simulink model "road_disturbances"  (R2020b)
settings: Solver=VariableStepAuto  StartTime=0.0  StopTime=10.0  MaxStep=1e-2  RelTol=1e-3
libraries: simulink x2
settings Model: Creator=kjartan  LastModifiedBy=kjartan

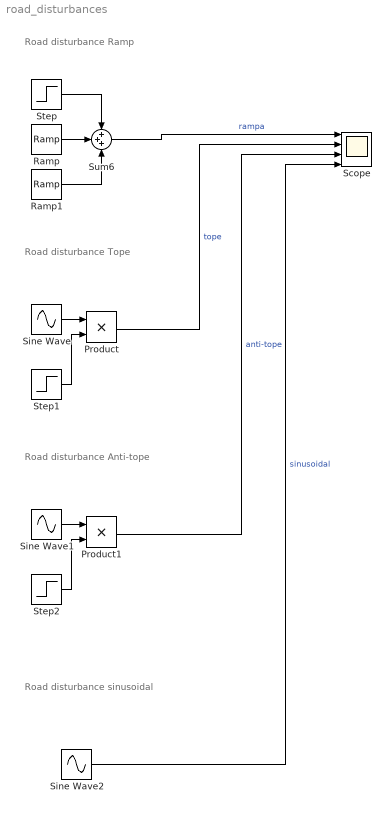
== system road_disturbances ==
  note: Road disturbance
      | Ramp
  note: Road disturbance
      | Tope
  note: Road disturbance
      | Anti-tope
  note: Road disturbance
      | sinusoidal
  Product : Product
  Product1 : Product
  Ramp : simulink/Sources/Ramp  slope=1  start=0  InitialOutput=0
  Ramp1 : simulink/Sources/Ramp  slope=-1  start=0.4  InitialOutput=0
  Scope : Scope  NumInputPorts=4
  Sine Wave : Sin  Amplitude=3  Bias=-sin(pi/3)*3  Frequency=2  Phase=pi/3  SampleTime=0
  Sine Wave1 : Sin  Amplitude=-3  Bias=sin(pi/3)*3  Frequency=2  Phase=pi/3  SampleTime=0
  Sine Wave2 : Sin  Amplitude=.05  Frequency=2*pi*10  SampleTime=0
  Step : Step  Time=.4  After=-0.4  SampleTime=0
  Step1 : Step  Time=2*pi/12  Before=1  After=0  SampleTime=0
  Step2 : Step  Time=2*pi/12  Before=1  After=0  SampleTime=0
  Sum6 : Sum  Inputs=+++
  wires:
  Ramp1/1 -> Sum6/3
  Ramp/1 -> Sum6/2
  Step/1 -> Sum6/1
  Sine Wave/1 -> Product/1
  Step1/1 -> Product/2
  Sum6/1 -> Scope/1  "rampa"
  Product/1 -> Scope/2  "tope"
  Step2/1 -> Product1/2
  Product1/1 -> Scope/3  "anti-tope"
  Sine Wave1/1 -> Product1/1
  Sine Wave2/1 -> Scope/4  "sinusoidal"
